simulink model "n1"  (R2021a)
settings: Solver=VariableStepAuto  StartTime=0.0  StopTime=10.0  RelTol=1e-3
undefined symbols (not defined in the file): Earth, WGS84
libraries: aerolibfltsims x2, shared6dof x1, aerolibanim x1, aerolibtransform2 x1
settings Model: Creator=samlo  LastModifiedBy=samlo

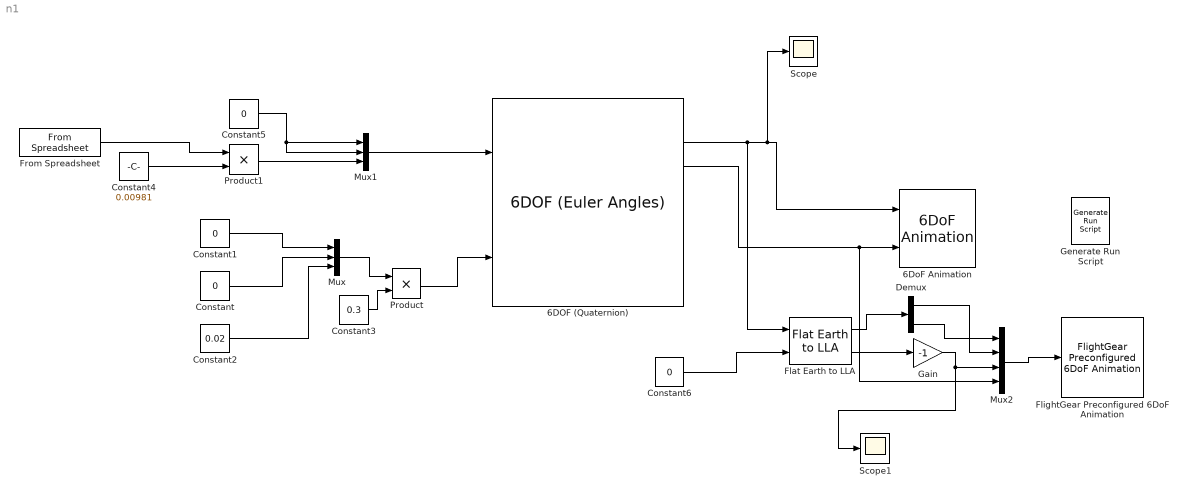
== system n1 ==
  6DOF (Quaternion) : shared6dof/6DOF (Euler Angles)  units=Metric (MKS)  mtype=Fixed  rep=Quaternion  xme_0=[0 0 0]  Vm_0=[0 0 0]  eul_0=[0 0 0]  pm_0=[0 0 0]  mass_0=1.187  mass_e=0.5  mass_f=2.0  inertia=eye(3)  inertia_e=eye(3)  inertia_f=2*eye(3)  k_quat=1.0  vre_flag=on  abi_flag=off  aMode=0  xme_statename=''  Vm_statename=''  eul_statename=''  quat_statename=''  pm_statename=''  mass_statename=''
      settings: SourceProductBaseCode=AE,PW,DR,MT,UV,VE
  6DoF Animation : aerolibanim/6DoF Animation  u1=[0 4000 -2000 2000 -5000 -3000]  u2=0.1  u3=1.0  u4=[4000 0 -5000]  u5=Fixed position  u6=[2000 500 -3150]  u7=10  u8=on
  Constant{,1,5..6} (4 alike) : Constant  Value=0
  Constant2 : Constant  Value=0.02
  Constant3 : Constant  Value=0.3
  Constant4 : Constant  Value=0.00981
  Demux : Demux  Outputs=2
  Flat Earth to LLA : aerolibtransform2/Flat Earth to LLA  units=Metric (MKS)  ptype=Earth (WGS84)  F=1/298.257223563  R=6378137  refPosPort=off  LL0=[0 10]  psi=0
  FlightGear Preconfigured 6DoF Animation : aerolibfltsims/FlightGear Preconfigured 6DoF Animation  xFlightGearVersion=v2019.1  DestinationIpAddress=127.0.0.1  DestinationPort=5502  SampleTime=1/30  packetVersion=24
  From Spreadsheet : FromSpreadsheet  FileName=v7.xlsx  TreatFirstColumnAs=Data  SampleTime=1.1
  Gain : Gain  Gain=-1
  Generate Run Script : aerolibfltsims/Generate Run Script  Architecture=Win64  dataFlow=Send  GeometryModelName=N11  AirportId=KSFO  RunwayId=10L  InitialAltitude=7224  InitialHeading=113  OffsetDistance=4.72  OffsetAzimuth=0  InstallScenery=off  DisableShaders=on  OriginAddress=127.0.0.1  DestinationPort=5502  OriginPort=5505  LocalAddress=127.0.0.1  OutputFileName=runfg.bat  FlightGearBaseDirectory=C:\Program Files\FlightGear 2020.3.6
  Mux : Mux  Inputs=3
  Mux1 : Mux  Inputs=3
  Mux2 : Mux
  Product : Product
  Product1 : Product
  Scope : Scope
  Scope1 : Scope
  wires:
  6DOF (Quaternion)/2 -> Flat Earth to LLA/1, Scope/1, 6DoF Animation/1
  6DOF (Quaternion)/3 -> Mux2/4, 6DoF Animation/2
  Constant1/1 -> Mux/1
  Constant/1 -> Mux/2
  Constant2/1 -> Mux/3
  Mux/1 -> Product/1
  Constant3/1 -> Product/2
  Mux1/1 -> 6DOF (Quaternion)/1
  From Spreadsheet/1 -> Product1/1
  Constant4/1 -> Product1/2
  Constant5/1 -> Mux1/2, Mux1/1
  Constant6/1 -> Flat Earth to LLA/2
  Mux2/1 -> FlightGear Preconfigured 6DoF Animation/1
  Flat Earth to LLA/1 -> Demux/1
  Demux/1 -> Mux2/2
  Demux/2 -> Mux2/1
  Flat Earth to LLA/2 -> Gain/1
  Product1/1 -> Mux1/3
  Gain/1 -> Scope1/1, Mux2/3
  Product/1 -> 6DOF (Quaternion)/2
